simulink model "LAB3_N1"  (R2023b)
settings: Solver=VariableStepAuto  StartTime=0.0  StopTime=30  RelTol=1e-3
settings Model: Creator=HP  LastModifiedBy=User

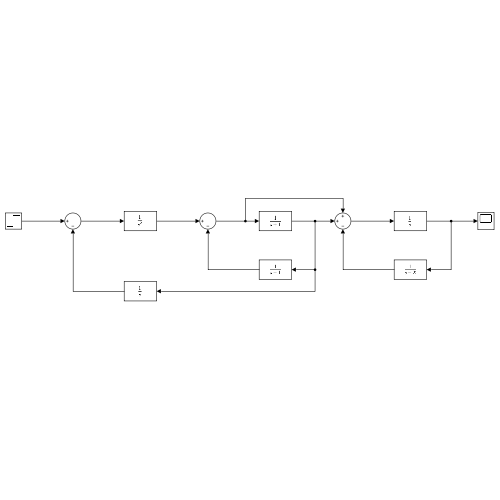
[thumbnail: Simulink's stored preview of the top-level diagram]
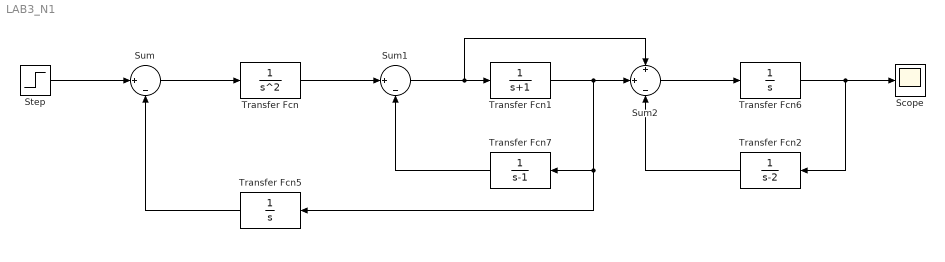
== system LAB3_N1 ==
  Scope : Scope
  Step : Step  SampleTime=0
  Sum : Sum  Inputs=||+|-
  Sum1 : Sum  Inputs=||+|-
  Sum2 : Sum  Inputs=+|+|-
  Transfer Fcn : TransferFcn  Denominator=[1 0 0]
  Transfer Fcn1 : TransferFcn  Denominator=[1 1]
  Transfer Fcn2 : TransferFcn  Denominator=[1 -2]
  Transfer Fcn5 : TransferFcn  Denominator=[1 0]
  Transfer Fcn6 : TransferFcn  Denominator=[1 0]
  Transfer Fcn7 : TransferFcn  Denominator=[1 -1]
  wires:
  Sum/1 -> Transfer Fcn/1
  Transfer Fcn5/1 -> Sum/2
  Transfer Fcn1/1 -> Sum2/2, Transfer Fcn7/1, Transfer Fcn5/1
  Transfer Fcn/1 -> Sum1/1
  Sum1/1 -> Sum2/1, Transfer Fcn1/1
  Sum2/1 -> Transfer Fcn6/1
  Transfer Fcn2/1 -> Sum2/3
  Transfer Fcn7/1 -> Sum1/2
  Transfer Fcn6/1 -> Scope/1, Transfer Fcn2/1
  Step/1 -> Sum/1
